simulink model "Trajectory_Implementation"  (R2023a)
settings: Solver=VariableStepAuto  StartTime=0.0  StopTime=10  MaxStep=0.05  RelTol=1e-3
libraries: dspinverses x1, DaVinci_Lib x1
settings Model: Creator=ASUS  LastModifiedBy=afons

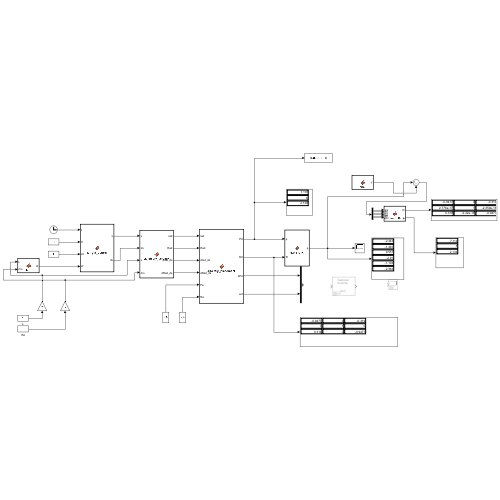
[thumbnail: Simulink's stored preview of the top-level diagram]
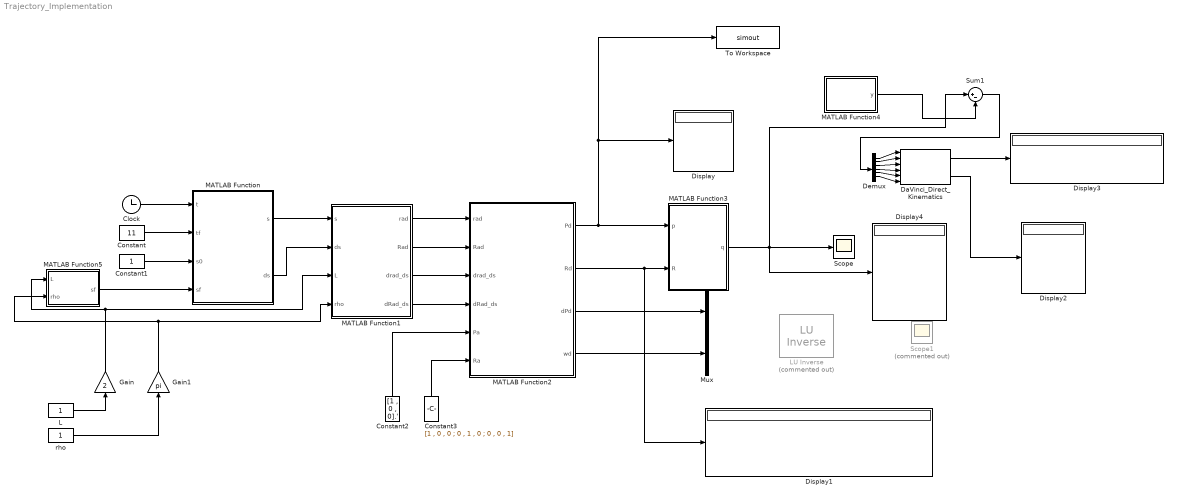
== system Trajectory_Implementation ==
  " LU Inverse" : dspinverses/ LU Inverse  Commented=on
  Clock : Clock
  Constant : Constant  Value=11
  Constant1 : Constant
  Constant2 : Constant  Value=[1 , 0 , 0].'
  Constant3 : Constant  Value=[1 , 0 , 0 ; 0 , 1 , 0 ; 0 , 0 , 1]
  DaVinci_Direct_Kinematics : DaVinci_Lib/DaVinci_Direct_Kinematics  SystemSampleTime=-1  VariantActivationTime=update diagram  Latency=0  AutoFrameSizeCalculation=off
      settings: LibrarySourceBlock=|
      | simulink/User-Defined
      | Functions/MATLAB Function
  Demux : Demux  Outputs=6
  Display{,1..4} (5 alike) : Display
  Gain : Gain  Gain=2
  Gain1 : Gain  Gain=pi
  L : Constant
  MATLAB Function : MATLAB Function  TreatAsAtomicUnit=on
  MATLAB Function1 : MATLAB Function  TreatAsAtomicUnit=on
  MATLAB Function2 : MATLAB Function  TreatAsAtomicUnit=on
  MATLAB Function3 : MATLAB Function  TreatAsAtomicUnit=on
  MATLAB Function4 : MATLAB Function  TreatAsAtomicUnit=on
  MATLAB Function5 : MATLAB Function  TreatAsAtomicUnit=on
  Mux : Mux  Inputs=2
  Scope : Scope
  Scope1 : Scope  Commented=on
  Sum1 : Sum  Inputs=|+-
  To Workspace : ToWorkspace  VariableName=simout  SaveFormat=Timeseries  SampleTime=-1
  rho : Constant
  wires:
  Constant1/1 -> MATLAB Function/3(s0)
  Constant/1 -> MATLAB Function/2(tf)
  Clock/1 -> MATLAB Function/1(t)
  Gain1/1 -> MATLAB Function5/2(rho), MATLAB Function1/4(rho)
  rho/1 -> Gain1/1
  L/1 -> Gain/1
  Gain/1 -> MATLAB Function5/1(L), MATLAB Function1/3(L)
  MATLAB Function/1(s) -> MATLAB Function1/1(s)
  MATLAB Function/2(ds) -> MATLAB Function1/2(ds)
  MATLAB Function1/1(rad) -> MATLAB Function2/1(rad)
  MATLAB Function1/2(Rad) -> MATLAB Function2/2(Rad)
  MATLAB Function1/3(drad_ds) -> MATLAB Function2/3(drad_ds)
  MATLAB Function1/4(dRad_ds) -> MATLAB Function2/4(dRad_ds)
  Constant2/1 -> MATLAB Function2/5(Pa)
  Constant3/1 -> MATLAB Function2/6(Ra)
  MATLAB Function2/1(Pd) -> To Workspace/1, Display/1, MATLAB Function3/1(p)
  MATLAB Function2/2(Rd) -> Display1/1, MATLAB Function3/2(R)
  MATLAB Function3/1(q) -> Display4/1, Scope/1, Sum1/1
  MATLAB Function2/3(dPd) -> Mux/1
  MATLAB Function2/4(wd) -> Mux/2
  Demux/6 -> DaVinci_Direct_Kinematics/6
  Demux/5 -> DaVinci_Direct_Kinematics/5
  Demux/4 -> DaVinci_Direct_Kinematics/4
  Demux/2 -> DaVinci_Direct_Kinematics/2
  Demux/3 -> DaVinci_Direct_Kinematics/3
  Demux/1 -> DaVinci_Direct_Kinematics/1
  DaVinci_Direct_Kinematics/2 -> Display2/1
  DaVinci_Direct_Kinematics/1 -> Display3/1
  MATLAB Function4/1(y) -> Sum1/2
  Sum1/1 -> Demux/1
  MATLAB Function5/1(sf) -> MATLAB Function/4(sf)

== matlab function Trajectory_Implementation/MATLAB Function1 ==
  data: s input; rad output; ds input; L input; rho input; Rad output; drad_ds output; dRad_ds output
function [rad,Rad,drad_ds,dRad_ds] = trajectory_velocity(s, ds, L, rho)

rad = zeros(3,1);
Rad = zeros(3,3);
drad_ds = zeros(3,1);
dRad_ds = zeros(3,3);

one = L;
two = L+rho*pi;
three = L+rho*pi+sqrt(L^2+4*rho^2);
four = L+2*rho*pi+sqrt(L^2+4*rho^2);
five = L+2*rho*pi+2*sqrt(L^2+4*rho^2);
six = L+3*rho*pi+2*sqrt(L^2+4*rho^2);
square = sqrt(L^2+4*rho^2);

if 0<=s && s<one

    rad=[0 s rho].';
    Rad=eye(3);
    drad_ds=[0 1 0].'*ds;
    dRad_ds=zeros(3)*ds;

elseif one<=s && s<two

    rad=[rho-rho*cos((s-one)/rho); L; rho-rho*sin((s-one)/rho)];
    Rad=[cos((s-one)/rho) 0 -sin((s-one)/rho);
                0         1         0        ;
         sin((s-one)/rho) 0 cos((s-one)/rho)];
    drad_ds=[sin((s-one)/rho); 0 ; -cos((s-one)/rho)]*ds;
    dRad_ds=[-sin((s-one)/rho)/rho 0 -cos((s-one)/rho)/rho;
                   0            0             0        ;
          cos((s-one)/rho)/rho  0 -sin((s-one)/rho)/rho]*ds;

elseif two<=s && s<three

    rad=[2*rho*(1-(s-two)/square); L*(1+(s-two)/square); rho];
    Rad=[-1  0  0;
          0  1  0;
          0  0 -1];
    drad_ds=[-2*rho/square; L/square ; 0]*ds;
    dRad_ds=zeros(3);

elseif three<=s && s<four

    rad=[rho-rho*cos((s-three)/rho); 2*L ; rho-rho*sin((s-three)/rho)];
    Rad=[-cos((s-three)/rho) 0 -sin((s-three)/rho);
                 0           1          0        ;
         -sin((s-three)/rho) 0 -cos((s-three)/rho)];
    drad_ds=[sin((s-three)/rho); 0 ; -cos((s-three)/rho)]*ds;
    dRad_ds=[sin((s-three)/rho)/rho 0 cos((s-three)/rho)/rho;
                    0            0              0        ;
         -cos((s-three)/rho)/rho 0 sin((s-three)/rho)/rho]*ds;

elseif four<=s && s<five

    rad=[2*rho*(1-(s-four)/square);L*(1+(s-four)/square);rho];
    Rad=eye(3);
    drad_ds=[-2*rho/square;L/square;0]*ds;
    dRad_ds=zeros(3);

elseif five<=s && s<six

    rad=[rho-rho*cos((s-five)/rho); 3*L ; rho-rho*sin((s-five)/rho)];
    Rad=[cos((s-five)/rho) 0 -sin((s-five)/rho);
                0          1          0        ;
         sin((s-five)/rho) 0 cos((s-five)/rho)];
    drad_ds=[sin((s-five)/rho);0;-cos((s-five)/rho)]*ds;
    dRad_ds=[-sin((s-five)/rho)/rho 0 -cos((s-five)/rho)/rho;
                    0            0              0        ;
          cos((s-five)/rho)/rho  0 -sin((s-five)/rho)/rho]*ds;

end

== matlab function Trajectory_Implementation/MATLAB Function ==
  data: t input; s output; tf input; s0 input; sf input; ds output
function [s,ds] = length_speed(t, tf, s0, sf)

s=0;
ds=0;

if 0<=t && t<=tf
    s=s0+3/(tf^2)*(sf-s0)*t^2-2/(tf^3)*(sf-s0)*t^3;
    ds=6/(tf^2)*(sf-s0)*t-6/(tf^3)*(sf-s0)*t^2;
else 
    s=sf;
    ds=0;
end

== matlab function Trajectory_Implementation/MATLAB Function2 ==
  data: rad input; Pd output; Rad input; drad_ds input; dRad_ds input; Rd output; dPd output; wd output; Pa input; Ra input
function [Pd,Rd,dPd,wd] = arbitrary_placement(rad,Rad,drad_ds,dRad_ds,Pa,Ra)

% %sem cross
Rd=Ra*Rad;
Pd=Pa+Ra*rad;
dPd=Ra*drad_ds;
w=dRad_ds*Rad'*Ra';
wd=[w(3,2);w(1,3);w(2,1)];


% %com cross?
% Rd=cross(Ra,Rad);
% Pd=Pa+cross(Ra,rad);
% dPd=cross(Ra,drad_ds);
% w=cross(cross(dRad_ds,Rad'),Ra');
% wd=[w(3,2);w(1,3);w(2,1)];

== matlab function Trajectory_Implementation/MATLAB Function3 ==
  data: p input; R input; q output
function q  = daVinciIK(p,R)
% IKin Calculations for DaVinci Robot
% q = [qx qy qz]

ii = [1 ; 0 ; 0];
jj = [0 ; 1 ; 0];
kk = [0 ; 0 ; 1];
a5 = .010;
a6 = .020;

x6 = R * ii;
y6 = R * jj;
z6 = R * kk;
p5 = p - a6 * x6;
z5 = z6;

z4 = cross(p5, z5) / norm(cross(p5, z5));
x5 = cross(z5, z4);
p3 = p5 - a5 * x5;

theta1 = atan2(-jj.' * p3, -ii.' * p3);
R1 = [cos(theta1) 0 -sin(theta1) ; sin(theta1) 0 cos(theta1) ; 0 -1 0];
x1 = R1 * ii;
y1 = R1 * jj;
z1 = cross(x1, y1);


theta2 = -atan2(-x1.' * p3, -y1.' * p3);
d3 = norm(p3);
z3 = p3 / norm(p3);
x4 = cross(z4, z3);
theta5 = -atan2(z5.' * x4, x5.' * x4);
y5 = cross(z5, x5);



theta6 = atan2(y5.' * x6, x5.' * x6);
R3 = [cos(theta1)*cos(theta2) , -sin(theta1) , cos(theta1)*sin(theta2) ; 
    sin(theta1) * cos(theta2) , cos(theta1) , sin(theta1) * sin(theta2) ; 
    -sin(theta2) , 0 , cos(theta2)];
x3 = R3 * ii;
y3 = R3 * jj;
theta4 = atan2(y3.' * x4, x3.' * x4);

q = [theta1 ; theta2 ; d3 ; theta4 ; theta5 ; theta6];

end

== matlab function Trajectory_Implementation/MATLAB Function4 ==
  data: y output
function y = fnc
%#codegen


y = [0 ; -pi/2 ; 0 ; pi/2 ; -pi/2 ; 0];

end

== matlab function Trajectory_Implementation/MATLAB Function5 ==
  data: L input; sf output; rho input
function sf = fcn(L,rho)


sf = L+3*rho*pi+2*sqrt(L^2+4*rho^2);
